simulink model "LOSdemoUKF"  (R2016b)
settings: Solver=FixedStepAuto  StartTime=0.0  StopTime=1200  FixedStep=0.1  RelTol=1e-3
settings Model: Creator=qys  LastModifiedBy=qys

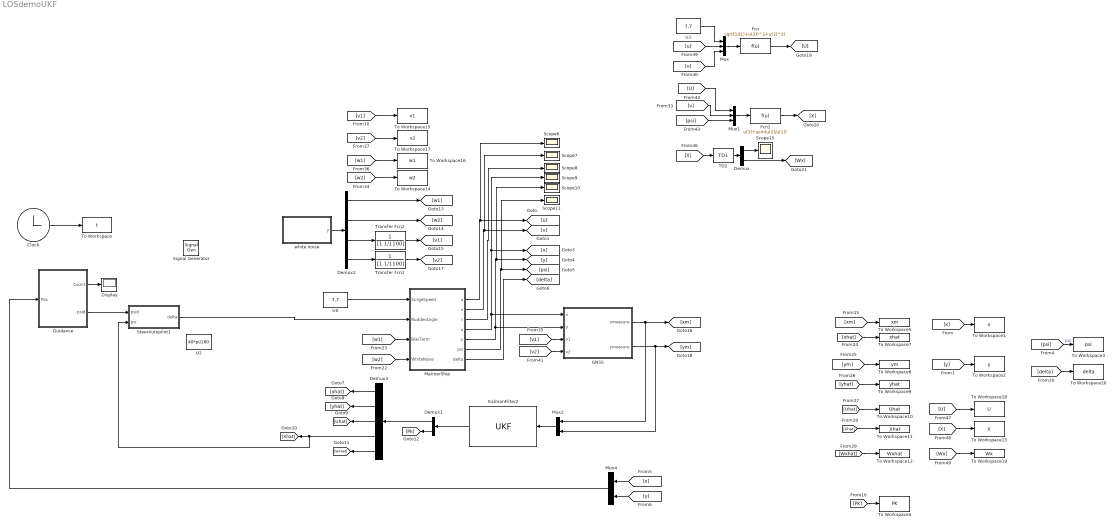
== system LOSdemoUKF ==
  Clock : Clock
  Demux : Demux  Outputs=2
  Demux1 : Demux  Outputs=[5 25]
  Demux2 : Demux
  Demux3 : Demux  Outputs=5
  Display : Display
  Fcn : Fcn  Expr=sqrt((u(1)+u(2))^2+u(3)^2)
  Fcn1 : Fcn  Expr=u(3)+asin(u(2)/u(1))
  GNSS : Subsystem
  Guidance : Subsystem  mask(Guidance){D=100, R=300, PointSet=[300 300 1500 300 2900 1900 2900 3900 1500 5500 300 5500]'}
      mask prompts: D "LookaheadDistance"; R "ChangeRadius"; PointSet "WayPointSet"
      mask help:
      | set lookahead distance\change radius\points number\points set
      | LookaheadDistance: D = 500
      | ChangeRadius: R = 300
      | WayPointSet: PointSet = [0 0 2900 2900 2900 4900 0 0 0 0]'
  KalmanFilter2 : S-Function  FunctionName=UKF  Parameters=Q,R  SFunctionDeploymentMode=off  EnableBusSupport=off  mask{Q=diag([1e-5 1e-5]), R=diag([0.1 0.1])}
      mask prompts: Q "Qk"; R "Rk"
      mask Display: disp('UKF')
  MarinerShip : Subsystem  mask(MarinerShip){InitialState=[0;0;0;100;300;0;0]}
      mask prompts: InitialState "initial state"
      mask help:
      | you can set ship initial state
      | x0 = [u;v;r;x;y;psi;delta]
      mask Display: disp('MainerShip')
  Mux : Mux  Inputs=3
  Mux1 : Mux  Inputs=3
  Mux2 : Mux  Inputs=2
  Mux4 : Mux  Inputs=2
  Scope{6..11,15} (7 alike) : Scope
  Signal Generator : SignalGenerator  WaveForm=square  Amplitude=40*pi/180  Frequency=0.005
  SteerAutopilot1 : Subsystem  mask(PID+TFF){Kp=1.45, Ti=1/100, Td=36.3}
      mask help:
      | TFF = T*Wxd/K+Wxd/K
      | PID = Kp*[(Xd-X)+Integrate(Xd-X)/Ti+Td*D(Xd-X)]
      | delta = TFF+PID*T/K
      | Kp = T*wn^2/K;
      | Td = T*(2*ksi*wn-1/T)/(K*Kp);
      | Ti = 10/wn;
  TD2 : S-Function  FunctionName=TD1  SFunctionDeploymentMode=off  EnableBusSupport=off
  To Workspace : ToWorkspace  VariableName=t  SampleTime=-1
  To Workspace1 : ToWorkspace  VariableName=x  SampleTime=-1
  To Workspace10 : ToWorkspace  VariableName=Uhat  SampleTime=-1
  To Workspace11 : ToWorkspace  VariableName=Xhat  SampleTime=-1
  To Workspace12 : ToWorkspace  VariableName=Wxhat  SampleTime=-1
  To Workspace13 : ToWorkspace  VariableName=X  SampleTime=-1
  To Workspace14 : ToWorkspace  VariableName=w2  SampleTime=-1
  To Workspace15 : ToWorkspace  VariableName=v1  SampleTime=-1
  To Workspace16 : ToWorkspace  VariableName=w1  SampleTime=-1
  To Workspace17 : ToWorkspace  VariableName=v2  SampleTime=-1
  To Workspace18 : ToWorkspace  VariableName=U  SampleTime=-1
  To Workspace19 : ToWorkspace  VariableName=Wx  SampleTime=-1
  To Workspace2 : ToWorkspace  VariableName=y  SampleTime=-1
  To Workspace20 : ToWorkspace  VariableName=delta  SampleTime=-1
  To Workspace3 : ToWorkspace  VariableName=psi  SampleTime=-1
  To Workspace4 : ToWorkspace  VariableName=PK  SampleTime=-1
  To Workspace5 : ToWorkspace  VariableName=xm  SampleTime=-1
  To Workspace7 : ToWorkspace  VariableName=xhat  SampleTime=-1
  To Workspace8 : ToWorkspace  VariableName=ym  SampleTime=-1
  To Workspace9 : ToWorkspace  VariableName=yhat  SampleTime=-1
  Transfer Fcn1 : TransferFcn  Denominator=[1 1/1100]
  Transfer Fcn2 : TransferFcn  Denominator=[1 1/1100]
  U0 : Constant  Value=7.7
  U1 : Constant  Value=7.7
  U2 : Constant  Value=40*pi/180
  white noise : MATLAB Function  TreatAsAtomicUnit=on
  wires:
  U0/1 -> MarinerShip/1(SurgeSpeed)
  Clock/1 -> To Workspace/1
  Demux1/1 -> Demux3/1
  Guidance/1(Count) -> Display/1
  MarinerShip/1(u) -> Scope6/1, [u]
  MarinerShip/2(v) -> Scope7/1, [v]
  MarinerShip/3(r) -> Scope8/1
  MarinerShip/4(x) -> [x], Scope9/1, GNSS/1(x)
  MarinerShip/5(y) -> Scope10/1, [y], GNSS/2(y)
  MarinerShip/6(psi) -> Scope11/1, [psi]
  MarinerShip/7(delta) -> [delta]
  [x] -> To Workspace1/1
  [y] -> To Workspace2/1
  [psi] -> To Workspace3/1  "psi"
  Demux3/1 -> [xhat]
  Demux3/2 -> [yhat]
  Demux3/3 -> [Uhat]
  Demux3/4 -> SteerAutopilot1/2(psi), [Xhat]
  Demux3/5 -> [Wxhat]
  [x] -> Mux4/1
  [y] -> Mux4/2
  Demux1/2 -> [Pk]
  [Pk] -> To Workspace4/1
  [delta] -> To Workspace20/1
  Demux2/2 -> [w2]
  [w2] -> MarinerShip/4(WhiteNoise)
  [w1] -> MarinerShip/3(BiasTerm)
  [w2] -> To Workspace14/1
  [w1] -> To Workspace16/1
  [v2] -> To Workspace17/1
  [u] -> Mux/2
  [v] -> Mux/3
  U1/1 -> Mux/1
  Mux/1 -> Fcn/1
  Fcn/1 -> [U]
  Demux2/1 -> [w1]
  [v1] -> To Workspace15/1
  [v1] -> GNSS/3(v1)
  [v2] -> GNSS/4(v2)
  GNSS/1(xmeasure) -> [xm], Mux2/1
  GNSS/2(ymeasure) -> Mux2/2, [ym]
  [xm] -> To Workspace5/1
  [xhat] -> To Workspace7/1
  [ym] -> To Workspace8/1
  [yhat] -> To Workspace9/1
  [Uhat] -> To Workspace10/1
  [Xhat] -> To Workspace11/1
  [Wxhat] -> To Workspace12/1
  Mux1/1 -> Fcn1/1
  [U] -> Mux1/1
  [v] -> Mux1/2
  [psi] -> Mux1/3
  Fcn1/1 -> [X]
  [X] -> To Workspace13/1
  [U] -> To Workspace18/1
  [X] -> TD2/1
  TD2/1 -> Demux/1
  Demux/2 -> [Wx]
  [Wx] -> To Workspace19/1
  Mux4/1 -> Guidance/1(Pos)
  Transfer Fcn1/1 -> [v2]
  Demux2/3 -> Transfer Fcn2/1
  Transfer Fcn2/1 -> [v1]
  Guidance/2(psid) -> SteerAutopilot1/1(psid)
  Demux2/4 -> Transfer Fcn1/1
  Mux2/1 -> KalmanFilter2/1
  KalmanFilter2/1 -> Demux1/1
  white noise/1(y) -> Demux2/1
  Demux/1 -> Scope15/1
  SteerAutopilot1/1(delta) -> MarinerShip/2(RudderAngle)

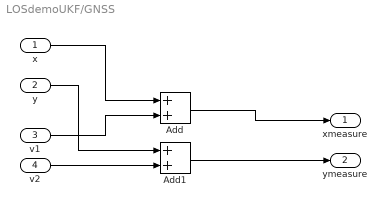
== system LOSdemoUKF/GNSS ==
  x : Inport
  y : Inport  Port=2
  v1 : Inport  Port=3
  v2 : Inport  Port=4
  Add : Sum
  Add1 : Sum
  xmeasure : Outport
  ymeasure : Outport  Port=2
  wires:
  x/1 -> Add/1
  v1/1 -> Add/2
  y/1 -> Add1/1
  v2/1 -> Add1/2
  Add/1 -> xmeasure/1
  Add1/1 -> ymeasure/1

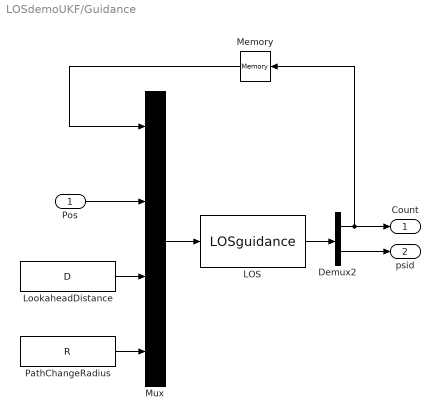
== system LOSdemoUKF/Guidance ==
  Pos : Inport
  Demux2 : Demux  Outputs=2
  LOS : S-Function  FunctionName=LOSguidance  Parameters=PointSet  SFunctionDeploymentMode=off  EnableBusSupport=off
  LookaheadDistance : Constant  Value=D
  Memory : Memory  X0=1
  Mux : Mux
  PathChangeRadius : Constant  Value=R
  Count : Outport
  psid : Outport  Port=2
  wires:
  LOS/1 -> Demux2/1
  Demux2/2 -> psid/1
  Pos/1 -> Mux/2
  LookaheadDistance/1 -> Mux/3
  PathChangeRadius/1 -> Mux/4
  Mux/1 -> LOS/1
  Demux2/1 -> Memory/1, Count/1
  Memory/1 -> Mux/1

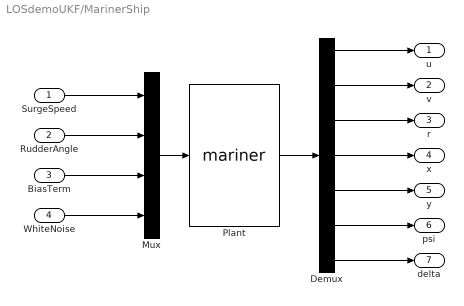
== system LOSdemoUKF/MarinerShip ==
  SurgeSpeed : Inport
  RudderAngle : Inport  Port=2
  BiasTerm : Inport  Port=3
  WhiteNoise : Inport  Port=4
  Demux : Demux  Outputs=7
  Mux : Mux
  Plant : S-Function  FunctionName=mariner  Parameters=InitialState  SFunctionDeploymentMode=off  EnableBusSupport=off
  u : Outport
  v : Outport  Port=2
  r : Outport  Port=3
  x : Outport  Port=4
  y : Outport  Port=5
  psi : Outport  Port=6
  delta : Outport  Port=7
  wires:
  SurgeSpeed/1 -> Mux/1
  RudderAngle/1 -> Mux/2
  BiasTerm/1 -> Mux/3
  WhiteNoise/1 -> Mux/4
  Mux/1 -> Plant/1
  Plant/1 -> Demux/1
  Demux/3 -> r/1
  Demux/4 -> x/1
  Demux/5 -> y/1
  Demux/6 -> psi/1
  Demux/7 -> delta/1
  Demux/2 -> v/1
  Demux/1 -> u/1

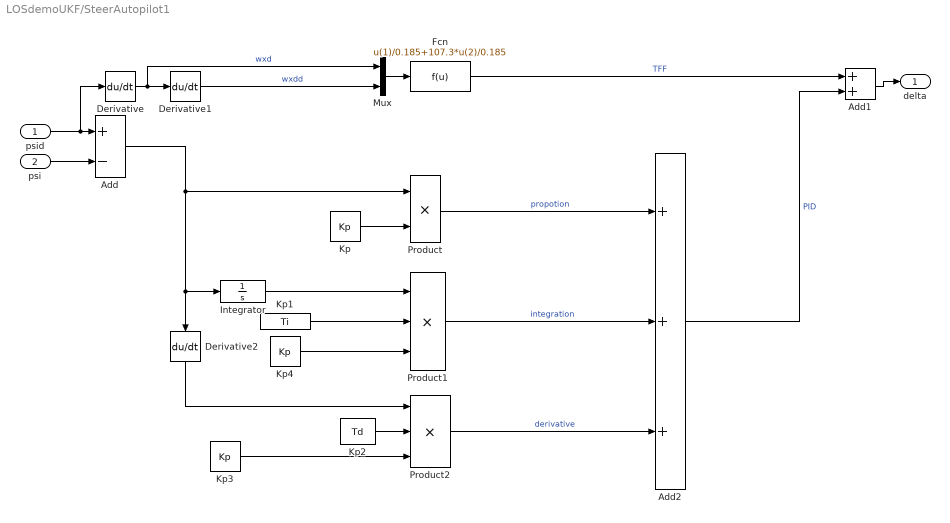
== system LOSdemoUKF/SteerAutopilot1 ==
  psid : Inport
  psi : Inport  Port=2
  Add : Sum  Inputs=+-
  Add1 : Sum
  Add2 : Sum  Inputs=+++
  Derivative : Derivative
  Derivative1 : Derivative
  Derivative2 : Derivative
  Fcn : Fcn  Expr=u(1)/0.185+107.3*u(2)/0.185
  Integrator : Integrator
  Kp : Constant  Value=Kp
  Kp1 : Constant  Value=Ti
  Kp2 : Constant  Value=Td
  Kp3 : Constant  Value=Kp
  Kp4 : Constant  Value=Kp
  Mux : Mux  Inputs=2
  Product : Product
  Product1 : Product  Inputs=3
  Product2 : Product  Inputs=3
  delta : Outport
  wires:
  psid/1 -> Derivative/1, Add/1
  psi/1 -> Add/2
  Derivative/1 -> Mux/1, Derivative1/1  "wxd"
  Derivative1/1 -> Mux/2  "wxdd"
  Mux/1 -> Fcn/1
  Fcn/1 -> Add1/1  "TFF"
  Add2/1 -> Add1/2  "PID"
  Add1/1 -> delta/1
  Kp/1 -> Product/2
  Kp1/1 -> Product1/2
  Integrator/1 -> Product1/1
  Derivative2/1 -> Product2/1
  Kp2/1 -> Product2/2
  Product/1 -> Add2/1  "propotion"
  Product1/1 -> Add2/2  "integration"
  Product2/1 -> Add2/3  "derivative"
  Add/1 -> Derivative2/1, Integrator/1, Product/1
  Kp3/1 -> Product2/3
  Kp4/1 -> Product1/3

== matlab function LOSdemoUKF/white noise ==
  data: y output
function y = fcn()
Qk = diag([1e-10 1e-10]);
Rk = diag([1e-1 1e-1]);
w = Qk*randn(2,1);
v = Rk*randn(2,1);
y = [w;v];
